simulink model "product_collapse_complex_test"  (Simulink 8.4)
settings: Solver=ode45  StartTime=0.0  StopTime=10.0  RelTol=1e-3
settings Model: Creator=arnaud  LastModifiedBy=arnaud
settings DataIOCC: SaveFormat=Structure

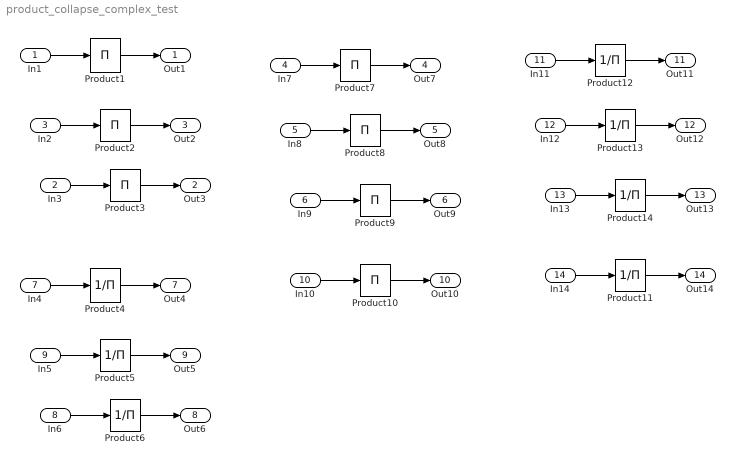
== system product_collapse_complex_test ==
  In1 : Inport
      settings: SignalType=complex
  In3 : Inport  Port=2  PortDimensions=[2 3]
      settings: SignalType=complex
  In2 : Inport  Port=3  PortDimensions=3
      settings: SignalType=complex
  In7 : Inport  Port=4
      settings: SignalType=complex
  In8 : Inport  Port=5  PortDimensions=3
      settings: SignalType=complex
  In9 : Inport  Port=6  PortDimensions=[2 3]
      settings: SignalType=complex
  In4 : Inport  Port=7
      settings: SignalType=complex
  In6 : Inport  Port=8  PortDimensions=[2 3]
      settings: SignalType=complex
  In5 : Inport  Port=9  PortDimensions=3
      settings: SignalType=complex
  In10 : Inport  Port=10  PortDimensions=[2 3]
      settings: SignalType=complex
  In11 : Inport  Port=11
      settings: SignalType=complex
  In12 : Inport  Port=12  PortDimensions=3
      settings: SignalType=complex
  In13 : Inport  Port=13  PortDimensions=[2 3]
      settings: SignalType=complex
  In14 : Inport  Port=14  PortDimensions=[2 3]
      settings: SignalType=complex
  Product1 : Product  Inputs=1  RndMeth=Zero
  Product10 : Product  Inputs=1  CollapseMode=Specified dimension  CollapseDim=2  RndMeth=Zero
  Product11 : Product  Inputs=/  CollapseMode=Specified dimension  CollapseDim=2  RndMeth=Zero
  Product12 : Product  Inputs=/  CollapseMode=Specified dimension  RndMeth=Zero
  Product13 : Product  Inputs=/  CollapseMode=Specified dimension  RndMeth=Zero
  Product14 : Product  Inputs=/  CollapseMode=Specified dimension  RndMeth=Zero
  Product2 : Product  Inputs=1  RndMeth=Zero
  Product3 : Product  Inputs=1  RndMeth=Zero
  Product4 : Product  Inputs=/  RndMeth=Zero
  Product5 : Product  Inputs=/  RndMeth=Zero
  Product6 : Product  Inputs=/  RndMeth=Zero
  Product7 : Product  Inputs=1  CollapseMode=Specified dimension  RndMeth=Zero
  Product8 : Product  Inputs=1  CollapseMode=Specified dimension  RndMeth=Zero
  Product9 : Product  Inputs=1  CollapseMode=Specified dimension  RndMeth=Zero
  Out1 : Outport
  Out3 : Outport  Port=2
  Out2 : Outport  Port=3
  Out7 : Outport  Port=4
  Out8 : Outport  Port=5
  Out9 : Outport  Port=6
  Out4 : Outport  Port=7
  Out6 : Outport  Port=8
  Out5 : Outport  Port=9
  Out10 : Outport  Port=10
  Out11 : Outport  Port=11
  Out12 : Outport  Port=12
  Out13 : Outport  Port=13
  Out14 : Outport  Port=14
  wires:
  In1/1 -> Product1/1
  Product1/1 -> Out1/1
  In3/1 -> Product3/1
  Product3/1 -> Out3/1
  In2/1 -> Product2/1
  Product2/1 -> Out2/1
  In7/1 -> Product7/1
  Product7/1 -> Out7/1
  In8/1 -> Product8/1
  Product8/1 -> Out8/1
  In9/1 -> Product9/1
  Product9/1 -> Out9/1
  In4/1 -> Product4/1
  Product4/1 -> Out4/1
  In6/1 -> Product6/1
  Product6/1 -> Out6/1
  In5/1 -> Product5/1
  Product5/1 -> Out5/1
  In10/1 -> Product10/1
  Product10/1 -> Out10/1
  In11/1 -> Product12/1
  Product12/1 -> Out11/1
  In12/1 -> Product13/1
  Product13/1 -> Out12/1
  In13/1 -> Product14/1
  Product14/1 -> Out13/1
  In14/1 -> Product11/1
  Product11/1 -> Out14/1
